simulink model "rov_sim"  (R2026a)
settings: Solver=FixedStepDiscrete  StopTime=t_max  FixedStep=ST
values from neighbouring files (symbols this model uses):
  P_bases_ned = [P_base1_ned'; P_base2_ned'; P_base3_ned'; P_base4_ned']    [sensors_auv.m]
  pos_ned = pos_ned + time * v_current    [trajectory_gen_cartesian.m]    (also in waypoints_gen.m = [pos_ned_n, pos_ned_e, pos_ned_d])
  Q = diag([repmat(q_pos,1,3), repmat(q_vel,1,3), repmat(q_euler,1,3), repmat(q_bias,1,3)])    [sensors_auv.m]
  R_ALG = R_ALG_base    [run_ablation.m]    (also in sensors_auv.m = diag([std_alg_rollpitch^2, std_alg_rollpitch^2, std_alg_yaw^)
  R_BO = R_BO_base    [run_ablation.m]    (also in sensors_auv.m = eye(N_bases) * (std_dev_BO^2))
  R_depth = std_dev_depth^2    (= 0.04)    [sensors_auv.m]
  rpy = zeros(length(time),3)    [trajectory_gen_cartesian.m]
  ST = 1/100    (= 0.01)    [waypoints_gen.m]
settings Model: Creator=39345  LastModifiedBy=39345

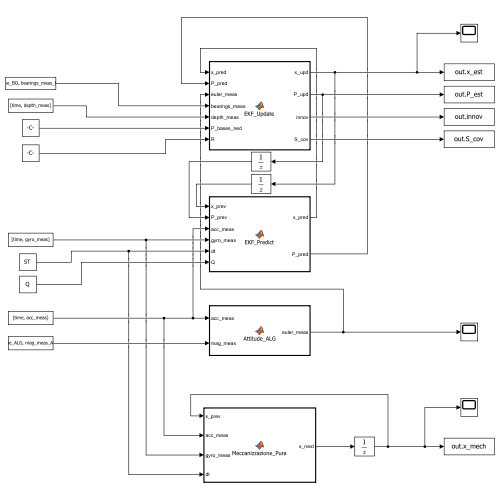
[thumbnail: Simulink's stored preview of the top-level diagram]
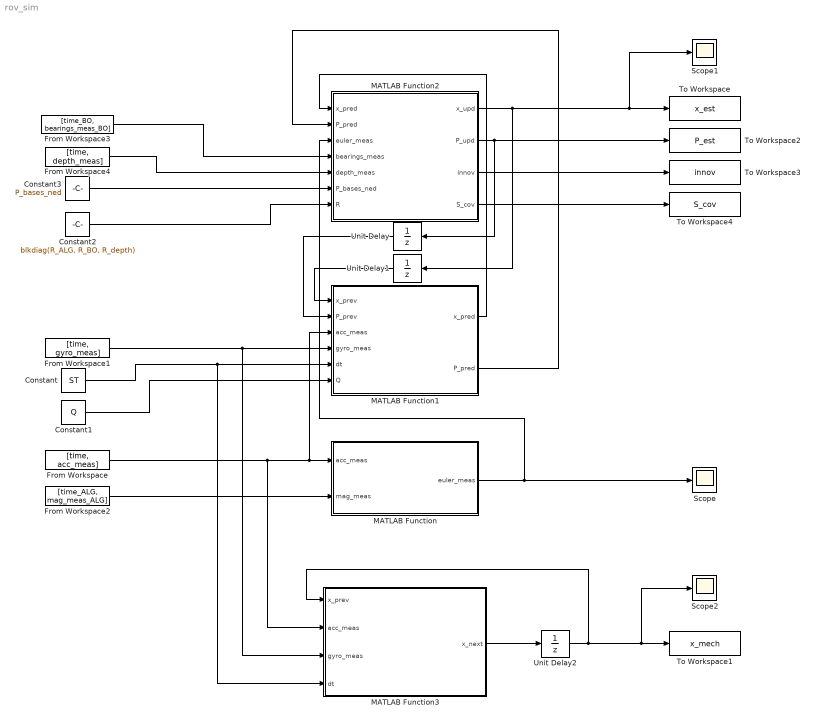
== system rov_sim ==
  Constant : Constant  Value=ST
  Constant1 : Constant  Value=Q
  Constant2 : Constant  Value=blkdiag(R_ALG, R_BO, R_depth)
  Constant3 : Constant  Value=P_bases_ned
  From Workspace : FromWorkspace  VariableName=[time, acc_meas]
  From Workspace1 : FromWorkspace  VariableName=[time, gyro_meas]
  From Workspace2 : FromWorkspace  VariableName=[time_ALG, mag_meas_ALG]
  From Workspace3 : FromWorkspace  VariableName=[time_BO, bearings_meas_BO]
  From Workspace4 : FromWorkspace  VariableName=[time, depth_meas]
  MATLAB Function : MATLAB Function  TreatAsAtomicUnit=on
  MATLAB Function1 : MATLAB Function  TreatAsAtomicUnit=on
  MATLAB Function2 : MATLAB Function  TreatAsAtomicUnit=on
  MATLAB Function3 : MATLAB Function  TreatAsAtomicUnit=on
  Scope : Scope
      settings: ActiveDisplayYMinimum=-1  ActiveDisplayYMaximum=1
  Scope1 : Scope
      settings: ActiveDisplayYMinimum=-1  ActiveDisplayYMaximum=1
  Scope2 : Scope
      settings: ActiveDisplayYMinimum=-1  ActiveDisplayYMaximum=1  DataLoggingVariableName=ScopeData2
  To Workspace : ToWorkspace  VariableName=x_est  SampleTime=-1
  To Workspace1 : ToWorkspace  VariableName=x_mech  SampleTime=-1
  To Workspace2 : ToWorkspace  VariableName=P_est  SampleTime=-1
  To Workspace3 : ToWorkspace  VariableName=innov  SampleTime=-1
  To Workspace4 : ToWorkspace  VariableName=S_cov  SampleTime=-1
  Unit Delay : UnitDelay  InitialCondition=eye(12)  SampleTime=-1
  Unit Delay1 : UnitDelay  InitialCondition=[pos_ned(1,:), 0, 0, 0, rpy(1,:), 0, 0, 0]'  SampleTime=-1
  Unit Delay2 : UnitDelay  InitialCondition=[pos_ned(1,:), 0, 0, 0, rpy(1,:)]'  SampleTime=-1
  wires:
  From Workspace/1 -> MATLAB Function3/2(acc_meas), MATLAB Function1/3(acc_meas), MATLAB Function/1(acc_meas)
  From Workspace2/1 -> MATLAB Function/2(mag_meas)
  From Workspace3/1 -> MATLAB Function2/4(bearings_meas)
  From Workspace1/1 -> MATLAB Function1/4(gyro_meas), MATLAB Function3/3(gyro_meas)
  MATLAB Function/1(euler_meas) -> Scope/1, MATLAB Function2/3(euler_meas)
  MATLAB Function1/1(x_pred) -> MATLAB Function2/1(x_pred)
  MATLAB Function1/2(P_pred) -> MATLAB Function2/2(P_pred)
  Constant1/1 -> MATLAB Function1/6(Q)
  Constant/1 -> MATLAB Function1/5(dt), MATLAB Function3/4(dt)
  Constant3/1 -> MATLAB Function2/6(P_bases_ned)
  Constant2/1 -> MATLAB Function2/7(R)
  MATLAB Function2/1(x_upd) -> Scope1/1, To Workspace/1, Unit Delay1/1
  MATLAB Function2/2(P_upd) -> Unit Delay/1, To Workspace2/1
  Unit Delay/1 -> MATLAB Function1/2(P_prev)
  Unit Delay1/1 -> MATLAB Function1/1(x_prev)
  MATLAB Function3/1(x_next) -> Unit Delay2/1
  Unit Delay2/1 -> Scope2/1, To Workspace1/1, MATLAB Function3/1(x_prev)
  From Workspace4/1 -> MATLAB Function2/5(depth_meas)
  MATLAB Function2/4(S_cov) -> To Workspace4/1
  MATLAB Function2/3(innov) -> To Workspace3/1

== matlab function rov_sim/MATLAB Function1 ==
  data: x_prev input; x_pred output; P_prev input; acc_meas input; gyro_meas input; dt input; Q input; P_pred output
function [x_pred, P_pred] = EKF_Predict(x_prev, P_prev, acc_meas, gyro_meas, dt, Q)
    % 1. Estrazione variabili di stato
    pos = x_prev(1:3);
    vel = x_prev(4:6);
    phi = x_prev(7); 
    theta = x_prev(8); 
    psi = x_prev(9);
    bg = x_prev(10:12);
    
    % 2. Matrici di Trasformazione Cinematica
    % Matrice di rotazione da Body a Nav
    C_b_n = [cos(theta)*cos(psi), sin(phi)*sin(theta)*cos(psi)-cos(phi)*sin(psi), cos(phi)*sin(theta)*cos(psi)+sin(phi)*sin(psi);
             cos(theta)*sin(psi), sin(phi)*sin(theta)*sin(psi)+cos(phi)*cos(psi), cos(phi)*sin(theta)*sin(psi)-sin(phi)*cos(psi);
             -sin(theta),         sin(phi)*cos(theta),                            cos(phi)*cos(theta)];
             
    % Matrice J per ratei di Eulero
    J = [1, sin(phi)*tan(theta), cos(phi)*tan(theta);
         0, cos(phi),           -sin(phi);
         0, sin(phi)/cos(theta), cos(phi)/cos(theta)];
         
    % 3. Equazioni Non Lineari della Dinamica
    omega_true = gyro_meas - bg; % Compensazione del bias stimato
    
    pos_dot = vel;
    vel_dot = C_b_n * acc_meas + [0; 0; 9.81];
    eta_dot = J * omega_true;
    bg_dot = [0; 0; 0];
    
    x_dot = [pos_dot; vel_dot; eta_dot; bg_dot];
    
    % Integrazione di Eulero al primo ordine
    x_pred = x_prev + x_dot * dt;
    x_pred(7:9) = wrapToPi(x_pred(7:9)); % Manteniamo gli angoli tra -pi e pi
    
    % 4. Calcolo della matrice Jacobiana F (12x12)
    F = eye(12);
    
    % Derivate della Posizione rispetto alla Velocità
    F(1:3, 4:6) = F(1:3, 4:6) + eye(3) * dt;
    
    % Derivate della Velocità rispetto all'Assetto (semplificate, dipendono da f^b)
    fx = acc_meas(1); fy = acc_meas(2); fz = acc_meas(3);
    
    % Elementi F(4:6, 7:9) - Jacobiana di (C_b_n * f^b) rispetto a phi, theta, psi
    F(4,7) = (cos(phi)*sin(theta)*cos(psi) + sin(phi)*sin(psi))*fy + (-sin(phi)*sin(theta)*cos(psi) + cos(phi)*sin(psi))*fz;
    F(4,8) = (-sin(theta)*cos(psi))*fx + (sin(phi)*cos(theta)*cos(psi))*fy + (cos(phi)*cos(theta)*cos(psi))*fz;
    F(4,9) = (-cos(theta)*sin(psi))*fx + (-sin(phi)*sin(theta)*sin(psi) - cos(phi)*cos(psi))*fy + (-cos(phi)*sin(theta)*sin(psi) + sin(phi)*cos(psi))*fz;
    
    F(5,7) = (cos(phi)*sin(theta)*sin(psi) - sin(phi)*cos(psi))*fy + (-sin(phi)*sin(theta)*sin(psi) - cos(phi)*cos(psi))*fz;
    F(5,8) = (-sin(theta)*sin(psi))*fx + (sin(phi)*cos(theta)*sin(psi))*fy + (cos(phi)*cos(theta)*sin(psi))*fz;
    F(5,9) = (cos(theta)*cos(psi))*fx + (sin(phi)*sin(theta)*cos(psi) - cos(phi)*sin(psi))*fy + (cos(phi)*sin(theta)*cos(psi) + sin(phi)*sin(psi))*fz;
    
    F(6,7) = (cos(phi)*cos(theta))*fy + (-sin(phi)*cos(theta))*fz;
    F(6,8) = (-cos(theta))*fx + (-sin(phi)*sin(theta))*fy + (-cos(phi)*sin(theta))*fz;
    F(6,9) = 0;
    
    % Moltiplichiamo per dt gli elementi della velocità
    F(4:6, 7:9) = F(4:6, 7:9) * dt;
    
    % Derivate dell'Assetto rispetto a se stesso (Jacobiana di J * omega)
    p = omega_true(1); q = omega_true(2); r = omega_true(3);
    F(7,7) = 1 + (cos(phi)*tan(theta)*q - sin(phi)*tan(theta)*r) * dt;
    F(7,8) = (sin(phi)/(cos(theta)^2)*q + cos(phi)/(cos(theta)^2)*r) * dt;
    F(8,7) = (-sin(phi)*q - cos(phi)*r) * dt;
    F(9,7) = (cos(phi)/cos(theta)*q - sin(phi)/cos(theta)*r) * dt;
    F(9,8) = (sin(phi)*sin(theta)/(cos(theta)^2)*q + cos(phi)*sin(theta)/(cos(theta)^2)*r) * dt;
    
    % Derivate dell'Assetto rispetto al Bias dei Giroscopi
    F(7:9, 10:12) = F(7:9, 10:12) - J * dt;
    
    % Propagazione della Covarianza
    P_pred = F * P_prev * F' + Q;
    
    % Simmetrizzazione per stabilità numerica
    P_pred = 0.5 * (P_pred + P_pred');
end

== matlab function rov_sim/MATLAB Function ==
  data: acc_meas input; euler_meas output; mag_meas input
function euler_meas = Attitude_ALG(acc_meas, mag_meas)
    % Estrazione componenti dai sensori
    fx = acc_meas(1);
    fy = acc_meas(2);
    fz = acc_meas(3);
    
    mx = mag_meas(1);
    my = mag_meas(2);
    mz = mag_meas(3);
    
    % 1. Calcolo Roll e Pitch dall'accelerometro
    % In condizioni di bassa dinamica l'accelerometro rileva la scomposizione della gravità
    roll = atan2(-fy, -fz);
    pitch = atan2(fx, sqrt(fy^2 + fz^2));
    
    % 2. Compensazione del tilt per il magnetometro
    % Proiettiamo il campo magnetico misurato in body frame sul piano orizzontale
    mx_h = mx * cos(pitch) + my * sin(pitch) * sin(roll) + mz * sin(pitch) * cos(roll);
    my_h = my * cos(roll) - mz * sin(roll);
    
    % 3. Calcolo dello Yaw
    yaw = atan2(-my_h, mx_h);
    
    % Output: vettore colonna [Roll; Pitch; Yaw]
    euler_meas = [roll; pitch; yaw];
end

== matlab function rov_sim/MATLAB Function2 ==
  data: x_pred input; x_upd output; P_pred input; euler_meas input; bearings_meas input; depth_meas input; P_bases_ned input; R input; P_upd output; innov output; S_cov output
function [x_upd, P_upd, innov, S_cov] = EKF_Update(x_pred, P_pred, euler_meas, bearings_meas, depth_meas, P_bases_ned, R)
    p_N = x_pred(1); p_E = x_pred(2); p_D = x_pred(3);
    
    num_boe = size(P_bases_ned, 1);
    num_meas = 3 + num_boe + 1; % 3 Eulero + N Bearing + 1 Profondità
    
    h_x = zeros(num_meas, 1);
    y   = zeros(num_meas, 1);
    
    % 1. Misure ALG
    h_x(1:3) = x_pred(7:9);
    y(1:3)   = euler_meas;
    
    % 2. Misure BO
    for i = 1:num_boe
        delta_N = P_bases_ned(i, 1) - p_N;
        delta_E = P_bases_ned(i, 2) - p_E;
        h_x(3 + i) = atan2(delta_E, delta_N);
        y(3 + i)   = bearings_meas(i);
    end
    
    % 3. Misura Profondità
    h_x(end) = p_D;
    y(end)   = depth_meas;
    
    innov = y - h_x;
    
    % Wrap angoli (NON wrappare la profondità all'ultimo indice!)
    for i = 1:(num_meas-1)
        innov(i) = wrapToPi(innov(i));
    end
    
    % Jacobiana H
    H = zeros(num_meas, 12);
    H(1:3, 7:9) = eye(3);
    
    for i = 1:num_boe
        delta_N = P_bases_ned(i, 1) - p_N;
        delta_E = P_bases_ned(i, 2) - p_E;
        dist_sq = delta_N^2 + delta_E^2;
        
        if dist_sq > 1e-4
            H(3 + i, 1) =  delta_E / dist_sq; 
            H(3 + i, 2) = -delta_N / dist_sq;
        end
    end
    
    H(end, 3) = 1; % Derivata Profondità
    
    % Update Kalman
    S_cov = H * P_pred * H' + R;
    K = P_pred * H' / S_cov;
    x_upd = x_pred + K * innov;
    x_upd(7:9) = wrapToPi(x_upd(7:9));
    
    P_upd = (eye(12) - K * H) * P_pred;
    P_upd = 0.5 * (P_upd + P_upd');
end

== matlab function rov_sim/MATLAB Function3 ==
  data: x_prev input; x_next output; acc_meas input; gyro_meas input; dt input
function x_next = Meccanizzazione_Pura(x_prev, acc_meas, gyro_meas, dt)
    % 1. Estrazione delle variabili di stato (9 componenti)
    pos   = x_prev(1:3);
    vel   = x_prev(4:6);
    phi   = x_prev(7); 
    theta = x_prev(8); 
    psi   = x_prev(9);
    
    % 2. Matrici di Trasformazione Cinematica
    % Matrice di rotazione da Body a Nav
    C_b_n = [cos(theta)*cos(psi), sin(phi)*sin(theta)*cos(psi)-cos(phi)*sin(psi), cos(phi)*sin(theta)*cos(psi)+sin(phi)*sin(psi);
             cos(theta)*sin(psi), sin(phi)*sin(theta)*sin(psi)+cos(phi)*cos(psi), cos(phi)*sin(theta)*sin(psi)-sin(phi)*cos(psi);
             -sin(theta),         sin(phi)*cos(theta),                            cos(phi)*cos(theta)];
             
    % Matrice J per ratei di Eulero
    J = [1, sin(phi)*tan(theta), cos(phi)*tan(theta);
         0, cos(phi),           -sin(phi);
         0, sin(phi)/cos(theta), cos(phi)/cos(theta)];
         
    % 3. Equazioni della Dinamica (Terra Piatta)[cite: 1]
    % Nota: Usiamo le misure grezze senza sottrarre il bias. Questo causa la deriva.
    pos_dot = vel;
    vel_dot = C_b_n * acc_meas + [0; 0; 9.81]; % Accelerazione cinematica + Gravità
    eta_dot = J * gyro_meas;
    
    % 4. Integrazione di Eulero al primo ordine
    pos_next = pos + pos_dot * dt;
    vel_next = vel + vel_dot * dt;
    eta_next = [phi; theta; psi] + eta_dot * dt;
    
    % Wrap degli angoli tra -pi e pi
    eta_next(1) = wrapToPi(eta_next(1));
    eta_next(2) = wrapToPi(eta_next(2));
    eta_next(3) = wrapToPi(eta_next(3));
    
    % 5. Composizione dello stato aggiornato
    x_next = [pos_next; vel_next; eta_next];
end
